simulink subsystem "active_infeed"  (R2023b)
settings: Solver=VariableStepAuto  StartTime=0.0  StopTime=10.0  RelTol=1e-3
model mask{P=0, Ts=0}
values from neighbouring files (symbols this model uses):
  Ts = ts(k)    [example_MW.m]
libraries: ee_lib x11, nesl_utility x10, fl_lib x4, eeTransforms x3, eeAdaptiveController x1, slpidlib x1, eeSinusoidalMeasurement x1, eeGeneralControl x1, eePwmGeneratorTwoLevel x1
settings Model: Creator=neugebch  LastModifiedBy=neugebch

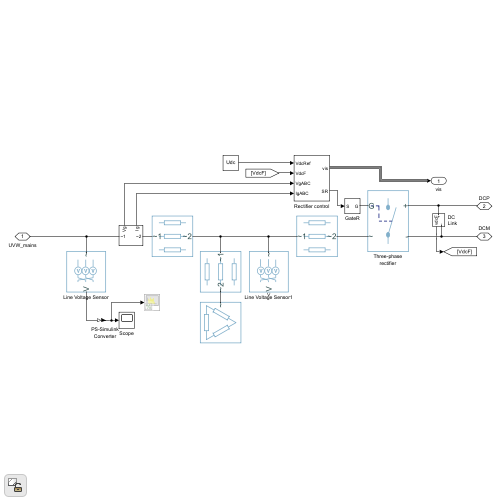
[thumbnail: Simulink's stored preview of the top-level diagram]
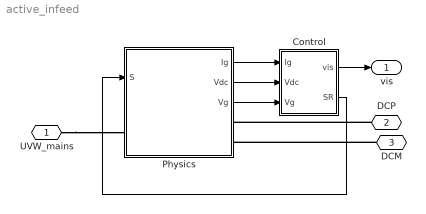
== system active_infeed ==
  Control : Subsystem
  Physics : Subsystem
  UVW_mains : PMIOPort  Side=Left
  DCP : PMIOPort  Port=2  Side=Right
  DCM : PMIOPort  Port=3  Side=Right
  vis : Outport
  wires:
  Physics/3(Vg) -> Control/3(Vg)
  Physics/2(Vdc) -> Control/2(Vdc)
  Physics/1(Ig) -> Control/1(Ig)
  Control/2(SR) -> Physics/1(S)
  Control/1(vis) -> vis/1
  connections:
  DCM/RConn1 -- Physics/RConn2
  UVW_mains/RConn1 -- Physics/LConn1
  DCP/RConn1 -- Physics/RConn1

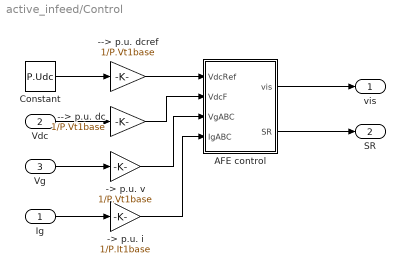
== system active_infeed/Control ==
  Ig : Inport
  Vdc : Inport  Port=2
  Vg : Inport  Port=3
  --> p.u. dc : Gain  Gain=1/P.Vt1base
  --> p.u. dcref : Gain  Gain=1/P.Vt1base
  -> p.u. i : Gain  Gain=1/P.It1base
  -> p.u. v : Gain  Gain=1/P.Vt1base
  AFE control : Subsystem
  Constant : Constant  Value=P.Udc
  vis : Outport
  SR : Outport  Port=2
  wires:
  --> p.u. dc/1 -> AFE control/2(VdcF)
  Vdc/1 -> --> p.u. dc/1
  --> p.u. dcref/1 -> AFE control/1(VdcRef)
  AFE control/2(SR) -> SR/1
  Ig/1 -> -> p.u. i/1
  AFE control/1(vis) -> vis/1
  Vg/1 -> -> p.u. v/1
  Constant/1 -> --> p.u. dcref/1
  -> p.u. v/1 -> AFE control/3(VgABC)
  -> p.u. i/1 -> AFE control/4(IgABC)

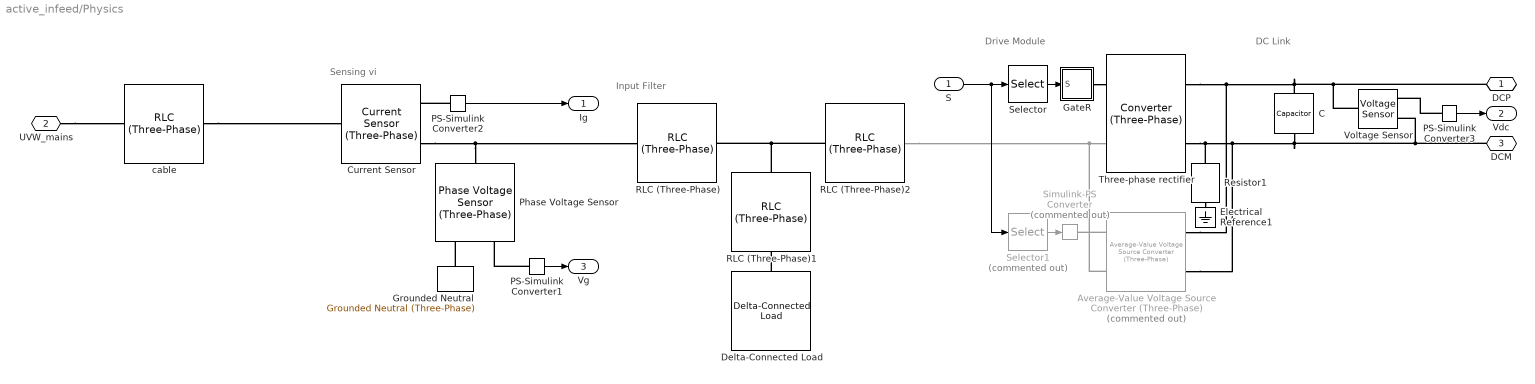
== system active_infeed/Physics ==
  note: Sensing vi
  note: Input Filter
  note: DC
      | Link
  note: Drive Module
  S : Inport
  Average-Value Voltage Source Converter (Three-Phase) : ee_lib/Semiconductors & Converters/Converters/Average-Value Voltage Source Converter (Three-Phase)  Commented=on  port_option=ee.enum.threePhasePort.composite  frequency_option=ee.enum.converters.frequency.constant  FRated=P.fn Hz  losses_parameterization=ee.enum.converters.losses.fixed  Pfixed=1 W  ks=0.01  kc1=1.7 V  kc2=0.01 Ohm  Ploss_vect=[100, 800, 1870, 3250, 4900] W  Irms_vect=[10, 100, 200, 300, 400] A  Vdc_nom=300 V  thermal_mass=30000 J/K  temperature_specify=off  temperature_priority=High  temperature=298.15 K  temperature_nominal_specify=off  temperature_nominal_unit=K  temperature_nominal_value=1
      settings: InternalSimscapePortConfiguration="{\"Bottom\":[],\"Left\":[{\"id\":\"ModWave\",\"label\":\"ModWave\",\"type\":\"input\"},{\"id\":\"N\",\"label\":\"~\",\"type\":\"foundation.electrical.three_phase\"}],\"Right\":[{\"id\":\"p\",\"label\":\"+\",\"type\":\"foundation.electrical.electrical\"},{\"id\":\"n\",\"label\":\"-\",\"type\":\"foundation.electrical.electrical\"}],\"Top\":[]}"
  C : fl_lib/Electrical/Electrical Elements/Capacitor  c=P.Cd F  r=P.Rd Ohm  g=1/P.Rd2 1/Ohm  i_specify=off  i_priority=None  i=0 A  i_nominal_specify=off  i_nominal_unit=A  i_nominal_value=1  v_specify=off  v_priority=None  v=0 V  v_nominal_specify=off  v_nominal_unit=V  v_nominal_value=1  vc_specify=on  vc_priority=None  vc=0 V  vc_nominal_specify=off  vc_nominal_unit=V  vc_nominal_value=1
  Current Sensor : ee_lib/Sensors & Transducers/Current Sensor (Three-Phase)
  Delta-Connected Load : ee_lib/Passive/RLC Assemblies/Delta-Connected Load  parameterization=ee.enum.rlc.parameterization.direct  component_structure=ee.enum.rlc.structure.C  component_structure_PQ=ee.enum.rlc.structure.SeriesRC  R=1 Ohm  L=1e-3 H  C=P.Cz F  VRated=24e3 V  FRated=60 Hz  P=1e3 W  Qpos=1e2 A*V  Qneg=-1e2 A*V  R_parasitic=0 Ohm  G_parasitic=0 1/Ohm  R_parasitic_PQ=0 Ohm  G_parasitic_PQ=0 1/Ohm  Vmag0=24e3 V  Vang0=0 deg  Freq0=60 Hz  IL_specify=off  IL_priority=High  IL=[0, 0, 0] A  IL_nominal_specify=off  IL_nominal_unit=A  IL_nominal_value=1  VC_specify=off  VC_priority=High  VC=[0, 0, 0] V  VC_nominal_specify=off  VC_nominal_unit=V  VC_nominal_value=1
      settings: InternalSimscapePortConfiguration="{\"Bottom\":[],\"Left\":[{\"id\":\"N\",\"label\":\"~\",\"type\":\"foundation.electrical.three_phase\"}],\"Right\":[],\"Top\":[]}"
  Electrical Reference1 : fl_lib/Electrical/Electrical Elements/Electrical Reference
  GateR : Subsystem
  Grounded Neutral : ee_lib/Connectors & References/Grounded Neutral (Three-Phase)
  PS-Simulink Converter1 : nesl_utility/PS-Simulink Converter  PhysicalDomain=network_engine_domain  SubClassName=ps_output  LeftPortType=input  RightPortType=output  PseudoPeriodic=off  Frequencies=[]  VectorFormat=1-D array  Unit=1  AffineConversion=off
  PS-Simulink Converter2 : nesl_utility/PS-Simulink Converter  PhysicalDomain=network_engine_domain  SubClassName=ps_output  LeftPortType=input  RightPortType=output  PseudoPeriodic=off  Frequencies=[]  VectorFormat=1-D array  Unit=1  AffineConversion=off
  PS-Simulink Converter3 : nesl_utility/PS-Simulink Converter  PhysicalDomain=network_engine_domain  SubClassName=ps_output  LeftPortType=input  RightPortType=output  PseudoPeriodic=off  Frequencies=[]  VectorFormat=1-D array  Unit=1  AffineConversion=off
  Phase Voltage Sensor : ee_lib/Sensors & Transducers/Phase Voltage Sensor (Three-Phase)
  RLC (Three-Phase) : ee_lib/Passive/RLC Assemblies/RLC (Three-Phase)  component_structure=ee.enum.rlc.structure.SeriesRL  R=P.Le*P.om/P.X_R_Le Ohm  L=P.Le H  C=1e-6 F  R_parasitic=0 Ohm  G_parasitic=0 1/Ohm  IL_specify=off  IL_priority=High  IL=[0, 0, 0] A  IL_nominal_specify=off  IL_nominal_unit=A  IL_nominal_value=1  VC_specify=off  VC_priority=High  VC=[0, 0, 0] V  VC_nominal_specify=off  VC_nominal_unit=V  VC_nominal_value=1
      settings: InternalSimscapePortConfiguration="{\"Bottom\":[],\"Left\":[{\"id\":\"N1\",\"label\":\"~1\",\"type\":\"foundation.electrical.three_phase\"}],\"Right\":[{\"id\":\"N2\",\"label\":\"~2\",\"type\":\"foundation.electrical.three_phase\"}],\"Top\":[]}"
  RLC (Three-Phase)1 : ee_lib/Passive/RLC Assemblies/RLC (Three-Phase)  component_structure=ee.enum.rlc.structure.R  R=P.Rz Ohm  L=1e-3 H  C=1e-6 F  R_parasitic=0 Ohm  G_parasitic=0 1/Ohm  IL_specify=off  IL_priority=High  IL=[0, 0, 0] A  IL_nominal_specify=off  IL_nominal_unit=A  IL_nominal_value=1  VC_specify=off  VC_priority=High  VC=[0, 0, 0] V  VC_nominal_specify=off  VC_nominal_unit=V  VC_nominal_value=1
      settings: InternalSimscapePortConfiguration="{\"Bottom\":[],\"Left\":[{\"id\":\"N1\",\"label\":\"~1\",\"type\":\"foundation.electrical.three_phase\"}],\"Right\":[{\"id\":\"N2\",\"label\":\"~2\",\"type\":\"foundation.electrical.three_phase\"}],\"Top\":[]}"
  RLC (Three-Phase)2 : ee_lib/Passive/RLC Assemblies/RLC (Three-Phase)  component_structure=ee.enum.rlc.structure.SeriesRL  R=P.Lk*P.om/P.X_R_Lk Ohm  L=P.Lk H  C=1e-6 F  R_parasitic=0 Ohm  G_parasitic=0 1/Ohm  IL_specify=off  IL_priority=High  IL=[0, 0, 0] A  IL_nominal_specify=off  IL_nominal_unit=A  IL_nominal_value=1  VC_specify=off  VC_priority=High  VC=[0, 0, 0] V  VC_nominal_specify=off  VC_nominal_unit=V  VC_nominal_value=1
      settings: InternalSimscapePortConfiguration="{\"Bottom\":[],\"Left\":[{\"id\":\"N1\",\"label\":\"~1\",\"type\":\"foundation.electrical.three_phase\"}],\"Right\":[{\"id\":\"N2\",\"label\":\"~2\",\"type\":\"foundation.electrical.three_phase\"}],\"Top\":[]}"
  Resistor1 : fl_lib/Electrical/Electrical Elements/Resistor  R=1e5 Ohm  i_specify=off  i_priority=None  i=0 A  i_nominal_specify=off  i_nominal_unit=A  i_nominal_value=1  v_specify=off  v_priority=None  v=0 V  v_nominal_specify=off  v_nominal_unit=V  v_nominal_value=1
  Selector : Selector  InputPortWidth=9  IndexOptions=Index vector (dialog)  Indices=1:6  OutputSizes=1
  Selector1 : Selector  Commented=on  InputPortWidth=9  IndexOptions=Index vector (dialog)  Indices=7:9  OutputSizes=1
  Simulink-PS Converter : nesl_utility/Simulink-PS Converter  Commented=on  PhysicalDomain=network_engine_domain  SubClassName=ps_input  LeftPortType=input  RightPortType=output  PseudoPeriodic=off  Frequencies=[]  NoiseDistribution=none  NoiseParameters=[]  Unit=1  AffineConversion=off  FilteringAndDerivatives=provide  SimscapeFilterOrder=1  InputFilterTimeConstant=0.001  UdotUserProvided=0
  Three-phase rectifier : ee_lib/Semiconductors & Converters/Converters/Converter (Three-Phase)  port_option=ee.enum.threePhasePort.composite  device_type=ee.enum.converters.switchingdevice.ideal  K=0  Vf=0.8 V  Ron=0.001 Ohm  Rds=0.001 Ohm  Goff=1e-5 1/Ohm  Vgt=1 V  Vgt_off=-1 V  Ih=1 A  Vth=0.5 V  diode_param=ee.enum.converters.protectiondiode.nodynamics  diode_Vf=0.8 V  diode_Ron=0.001 Ohm  diode_Goff=1e-5 1/Ohm  diode_C=50 nF  diode_iRM=-235 A  diode_iF=300 A  diode_idot=-50 A/us  diode_trr_param=ee.enum.converters.diodetrr.trr_factor  diode_trr_factor=3  diode_trr=15 us  diode_Qrr=1.5e+3 s*uA  snubber_type=ee.enum.converters.snubber.exclude  Cs=1e-5 F  Rs=1e-3 Ohm
  Voltage Sensor : fl_lib/Electrical/Electrical Sensors/Voltage Sensor
  cable : ee_lib/Passive/RLC Assemblies/RLC (Three-Phase)  component_structure=ee.enum.rlc.structure.SeriesRL  R=P.cab.l*P.cab.rl Ohm  L=P.cab.l*P.cab.ll H  C=1e-6 F  R_parasitic=0 Ohm  G_parasitic=0 1/Ohm  IL_specify=off  IL_priority=High  IL=[0, 0, 0] A  IL_nominal_specify=off  IL_nominal_unit=A  IL_nominal_value=1  VC_specify=off  VC_priority=High  VC=[0, 0, 0] V  VC_nominal_specify=off  VC_nominal_unit=V  VC_nominal_value=1
      settings: InternalSimscapePortConfiguration="{\"Bottom\":[],\"Left\":[{\"id\":\"N1\",\"label\":\"~1\",\"type\":\"foundation.electrical.three_phase\"}],\"Right\":[{\"id\":\"N2\",\"label\":\"~2\",\"type\":\"foundation.electrical.three_phase\"}],\"Top\":[]}"
  DCP : PMIOPort  Side=Right
  UVW_mains : PMIOPort  Port=2  Side=Left
  DCM : PMIOPort  Port=3  Side=Right
  Ig : Outport
  Vdc : Outport  Port=2
  Vg : Outport  Port=3
  wires:
  Selector1/1 -> Simulink-PS Converter/1
  Selector/1 -> GateR/1(S)
  PS-Simulink Converter3/1 -> Vdc/1
  PS-Simulink Converter2/1 -> Ig/1
  PS-Simulink Converter1/1 -> Vg/1
  S/1 -> Selector/1, Selector1/1
  connections:
  cable/RConn1 -- Current Sensor/LConn1
  Average-Value Voltage Source Converter (Three-Phase)/LConn1 -- Simulink-PS Converter/RConn1
  Resistor1/RConn1 -- Electrical Reference1/LConn1
  UVW_mains/RConn1 -- cable/LConn1
  PS-Simulink Converter3/LConn1 -- Voltage Sensor/RConn1
  Average-Value Voltage Source Converter (Three-Phase)/LConn2 -- Three-phase rectifier/LConn2 -- RLC (Three-Phase)2/RConn1
  GateR/RConn1 -- Three-phase rectifier/LConn1
  DCP/RConn1 -- Voltage Sensor/LConn1 -- C/LConn1 -- Average-Value Voltage Source Converter (Three-Phase)/RConn1 -- Three-phase rectifier/RConn1
  RLC (Three-Phase)/RConn1 -- RLC (Three-Phase)1/LConn1 -- RLC (Three-Phase)2/LConn1
  Phase Voltage Sensor/LConn1 -- RLC (Three-Phase)/LConn1 -- Current Sensor/RConn2
  PS-Simulink Converter2/LConn1 -- Current Sensor/RConn1
  Voltage Sensor/RConn2 -- DCM/RConn1 -- C/RConn1 -- Average-Value Voltage Source Converter (Three-Phase)/RConn2 -- Resistor1/LConn1 -- Three-phase rectifier/RConn2
  Grounded Neutral/LConn1 -- Phase Voltage Sensor/RConn2
  PS-Simulink Converter1/LConn1 -- Phase Voltage Sensor/RConn1
  Delta-Connected Load/LConn1 -- RLC (Three-Phase)1/RConn1

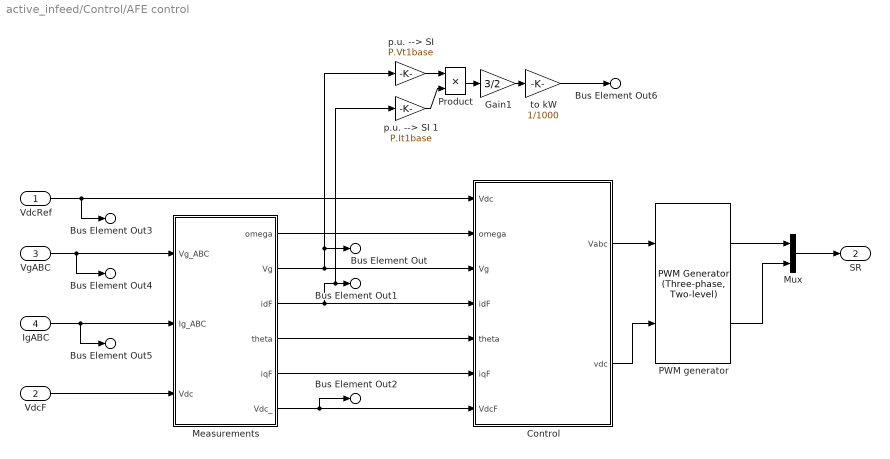
== system active_infeed/Control/AFE control ==
  VdcRef : Inport
  VdcF : Inport  Port=2
  VgABC : Inport  Port=3
  IgABC : Inport  Port=4
  Control : Subsystem
  Gain1 : Gain  Gain=3/2
  Measurements : Subsystem
  Mux : Mux  Inputs=2
  PWM generator : eePwmGeneratorTwoLevel/PWM Generator (Three-phase, Two-level)  PWMMode=Continuous PWM (CPWM)  CPWMMode=SVM: space vector modulation  DPWMMode=60 DPWM: 60 degree discontinuous PWM  fsw=P.fsw  Ts=Ts
  Product : Product
  p.u. --> SI : Gain  Gain=P.Vt1base
  p.u. --> SI 1 : Gain  Gain=P.It1base
  to kW : Gain  Gain=1/1000
  Bus Element Out : Outport  PortName=vis  Element=Vg
  Bus Element Out1 : Outport  PortName=vis  Element=idF
  Bus Element Out2 : Outport  PortName=vis  Element=VdcF
  Bus Element Out3 : Outport  PortName=vis  Element=VdcRef
  Bus Element Out4 : Outport  PortName=vis  Element=VgABC
  Bus Element Out5 : Outport  PortName=vis  Element=IgABC
  Bus Element Out6 : Outport  PortName=vis  Element=Pt
  SR : Outport  Port=2  VectorParamsAs1DForOutWhenUnconnected=off
  wires:
  Mux/1 -> SR/1
  PWM generator/1 -> Mux/1
  Control/2(vdc) -> PWM generator/2
  Control/1(Vabc) -> PWM generator/1
  PWM generator/2 -> Mux/2
  Measurements/6(Vdc_) -> Control/7(VdcF), Bus Element Out2/1
  VdcF/1 -> Measurements/3(Vdc)
  to kW/1 -> Bus Element Out6/1
  Measurements/3(idF) -> Control/4(idF), Bus Element Out1/1, p.u. --> SI 1/1
  Gain1/1 -> to kW/1
  p.u. --> SI/1 -> Product/1
  p.u. --> SI 1/1 -> Product/2
  Product/1 -> Gain1/1
  Measurements/2(Vg) -> Control/3(Vg), p.u. --> SI/1, Bus Element Out/1
  VdcRef/1 -> Bus Element Out3/1, Control/1(Vdc)
  Measurements/5(iqF) -> Control/6(iqF)
  Measurements/4(theta) -> Control/5(theta)
  Measurements/1(omega) -> Control/2(omega)
  IgABC/1 -> Measurements/2(Ig_ABC), Bus Element Out5/1
  VgABC/1 -> Measurements/1(Vg_ABC), Bus Element Out4/1

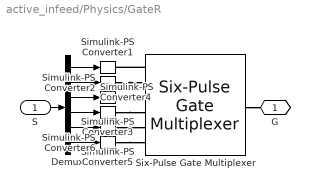
== system active_infeed/Physics/GateR ==
  S : Inport
  Demux : Demux  Outputs=6
  Simulink-PS Converter{1..6} (6 alike) : nesl_utility/Simulink-PS Converter  PhysicalDomain=network_engine_domain  SubClassName=ps_input  LeftPortType=input  RightPortType=output  PseudoPeriodic=off  Frequencies=[]  NoiseDistribution=none  NoiseParameters=[]  Unit=1  AffineConversion=off  FilteringAndDerivatives=zero  SimscapeFilterOrder=1  InputFilterTimeConstant=0.001  UdotUserProvided=1
  Six-Pulse Gate Multiplexer : ee_lib/Semiconductors & Converters/Converters/Six-Pulse Gate Multiplexer  port_option=ee.enum.controlport.ps
  G : PMIOPort  Side=Right
  wires:
  Demux/3 -> Simulink-PS Converter3/1
  Demux/6 -> Simulink-PS Converter6/1
  Demux/5 -> Simulink-PS Converter5/1
  S/1 -> Demux/1
  Demux/2 -> Simulink-PS Converter2/1
  Demux/1 -> Simulink-PS Converter1/1
  Demux/4 -> Simulink-PS Converter4/1
  connections:
  Six-Pulse Gate Multiplexer/RConn1 -- G/RConn1
  Six-Pulse Gate Multiplexer/LConn1 -- Simulink-PS Converter1/RConn1
  Simulink-PS Converter5/RConn1 -- Six-Pulse Gate Multiplexer/LConn5
  Simulink-PS Converter6/RConn1 -- Six-Pulse Gate Multiplexer/LConn6
  Simulink-PS Converter3/RConn1 -- Six-Pulse Gate Multiplexer/LConn3
  Simulink-PS Converter2/RConn1 -- Six-Pulse Gate Multiplexer/LConn2
  Simulink-PS Converter4/RConn1 -- Six-Pulse Gate Multiplexer/LConn4

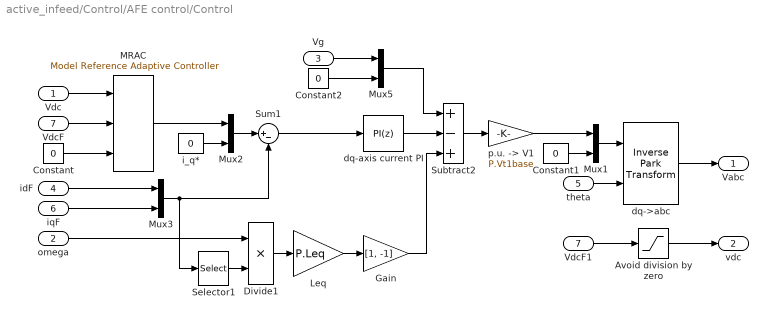
== system active_infeed/Control/AFE control/Control ==
  Vdc : Inport
  omega : Inport  Port=2
  Vg : Inport  Port=3
  idF : Inport  Port=4
  theta : Inport  Port=5
  iqF : Inport  Port=6
  VdcF : Inport  Port=7
  Avoid division by zero : Saturate  UpperLimit=1e6  LowerLimit=10
  Constant : Constant  Value=0
  Constant1 : Constant  Value=0  SampleTime=P.Tsc
  Constant2 : Constant  Value=0
  Divide1 : Product  Inputs=**
  Gain : Gain  Gain=[1, -1]
  Leq : Gain  Gain=P.Leq
  MRAC : eeAdaptiveController/Model Reference Adaptive Controller  Kp=P.Kp_vdc  Ki=P.Ki_vdc  Kd=0  Kaw=1000  UseFilter=off  N=100  up=5  lo=-5  Ts=P.Tsc  TfType=Discrete-time  numd=P.numd  dend=P.dend  numc=[1 1]  denc=[1 2 1]  Tsd=0.01  gamma=0.8
  Mux{1..3,5} (4 alike) : Mux  Inputs=2
  Selector1 : Selector  InputPortWidth=2  IndexOptions=Index vector (dialog)  Indices=[2 1]  OutputSizes=1
  Subtract2 : Sum  Inputs=+-+
  Sum1 : Sum  Inputs=|+-
  VdcF1 : InportShadow  Port=7
  dq->abc : eeTransforms/Inverse Park Transform  AxisAlignment=Q-axis  PowerInvariant=off
  dq-axis current PI : slpidlib/PID Controller  Controller=PI  Form=Parallel  TimeDomain=Discrete-time  UseExternalTs=off  SampleTime=P.Tsc  IntegratorMethod=Forward Euler  FilterMethod=Forward Euler  ControllerParametersSource=internal  P=[P.Kp_id, P.Kp_iq]  I=[P.Ki_id, P.Ki_iq]  UseKiTs=off  D=0  N=100  UseFilter=on  TunerSelectOption=Transfer Function Based (PID Tuner App)  InitialConditionSource=internal  InitialConditionForIntegrator=0  InitialConditionForFilter=0  DifferentiatorICPrevScaledInput=0  ExternalReset=none  TrackingMode=off  Kt=1  LimitOutput=on  SatLimitsSource=internal  UpperSaturationLimit=P.Req*1*10  LowerSaturationLimit=-P.Req*1*10  LinearizeAsGain=on  AntiWindupMode=back-calculation  Kb=1000  LimitIntegrator=off  UpperIntegratorSaturationLimit=inf  LowerIntegratorSaturationLimit=-inf  POutMin=[]  POutMax=[]  IOutMin=[]  IOutMax=[]  DOutMin=[]  DOutMax=[]  NOutMin=[]  NOutMax=[]  SumOutMin=[]  SumOutMax=[]  SaturationOutMin=[]  SaturationOutMax=[]  PParamMin=[]  PParamMax=[]  IParamMin=[]  IParamMax=[]  DParamMin=[]  DParamMax=[]  NParamMin=[]  NParamMax=[]  KbParamMin=[]  KbParamMax=[]  KtParamMin=[]  KtParamMax=[]  KbOutMin=[]  KbOutMax=[]  KtOutMin=[]  KtOutMax=[]  IntegratorOutMin=[]  IntegratorOutMax=[]  FilterOutMin=[]  FilterOutMax=[]  SumI1OutMin=[]  SumI1OutMax=[]  SumI2OutMin=[]  SumI2OutMax=[]  SumI3OutMin=[]  SumI3OutMax=[]  SumI4OutMin=[]  SumI4OutMax=[]  SumDOutMin=[]  SumDOutMax=[]  DifferentiatorOutMin=[]  DifferentiatorOutMax=[]  FilterDiffOutCoefMin=[]  FilterDiffOutCoefMax=[]  ReciprocalOutMin=[]  ReciprocalOutMax=[]  SumDenOutMin=[]  SumDenOutMax=[]  SumNumOutMin=[]  SumNumOutMax=[]  DivideOutMin=[]  DivideOutMax=[]  UdiffTsProdOutMin=[]  UdiffTsProdOutMax=[]  NTsProdOutMin=[]  NTsProdOutMax=[]  UintegralTsProdOutMin=[]  UintegralTsProdOutMax=[]  UngainTsProdOutMin=[]  UngainTsProdOutMax=[]  ClampingZeroOutDataTypeStr=Inherit: Inherit via back propagation  ClampingZeroOutMin=[]  ClampingZeroOutMax=[]  FilterDenConstantOutDataTypeStr=Inherit: Inherit via back propagation  FilterDenConstantOutMin=[]  FilterDenConstantOutMax=[]  PCopyOutDataTypeStr=Inherit: Inherit via back propagation  PCopyOutMin=[]  PCopyOutMax=[]  NCopyOutDataTypeStr=Inherit: Inherit via back propagation  NCopyOutMin=[]  NCopyOutMax=[]  IntegratorContinuousStateAttributes=''  IntegratorStateMustResolveToSignalObject=off  IntegratorRTWStateStorageClass=Auto  FilterContinuousStateAttributes=''  FilterStateMustResolveToSignalObject=off  FilterRTWStateStorageClass=Auto  ParallelPVariant=InternalParameters  IdealPVariant=Disabled  IVariant=InternalParameters  DVariant=Disabled  IntegratorVariant=Discrete  SatVariant=Enabled  AWVariant=BackCalculation  PCopyVariant=Disabled  TRVariant=Disabled  FdbkBlocksVariant=Forward  IdealPFdbkVariant=Disabled  SatFdbkVariant=Disabled  DerivativeFilterVariant=Disabled  NVariant=Disabled  NCopyVariant=Disabled_SignalSpec  FilterICVariant=Disabled  IntegratorICVariant=InternalICs  ExternalResetVariant=Disabled  TRSumVariant=Passthrough  SumFdbkVariant=Disabled  SumVariant=Sum_PI  TsampFilterVariant=InternalTs  TsampNgainVariant=Passthrough  TsampIntegralVariant=Disabled_SignalSpec  ExternalSaturationOutDataTypeStr=Inherit: Same as second input
  i_q* : Constant  Value=0
  "p.u. -> V1" : Gain  Gain=P.Vt1base
  Vabc : Outport
  vdc : Outport  Port=2
  wires:
  "p.u. -> V1"/1 -> Mux1/1
  Selector1/1 -> Divide1/2
  Gain/1 -> Subtract2/3
  Constant2/1 -> Mux5/2
  Mux5/1 -> Subtract2/1
  Vg/1 -> Mux5/1
  dq-axis current PI/1 -> Subtract2/2
  Sum1/1 -> dq-axis current PI/1
  Mux3/1 -> Selector1/1, Sum1/2
  Mux2/1 -> Sum1/1
  Leq/1 -> Gain/1
  Divide1/1 -> Leq/1
  MRAC/1 -> Mux2/1
  Constant/1 -> MRAC/3
  VdcF/1 -> MRAC/2
  Vdc/1 -> MRAC/1
  VdcF1/1 -> Avoid division by zero/1
  iqF/1 -> Mux3/2
  dq->abc/1 -> Vabc/1
  idF/1 -> Mux3/1
  Constant1/1 -> Mux1/2
  Mux1/1 -> dq->abc/1
  Subtract2/1 -> "p.u. -> V1"/1
  omega/1 -> Divide1/1
  i_q*/1 -> Mux2/2
  Avoid division by zero/1 -> vdc/1
  theta/1 -> dq->abc/2

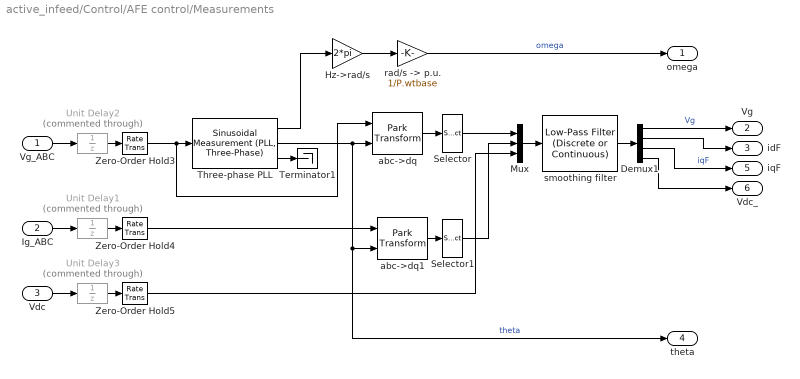
== system active_infeed/Control/AFE control/Measurements ==
  Vg_ABC : Inport
  Ig_ABC : Inport  Port=2
  Vdc : Inport  Port=3
  Demux1 : Demux
  Hz->rad/s : Gain  Gain=2*pi
  Mux : Mux  Inputs=3
  Selector : Selector  InputPortWidth=3  IndexOptions=Index vector (dialog)  Indices=[1]  OutputSizes=1
  Selector1 : Selector  InputPortWidth=3  IndexOptions=Index vector (dialog)  Indices=[1 2]  OutputSizes=1
  Terminator1 : Terminator
  Three-phase PLL : eeSinusoidalMeasurement/Sinusoidal Measurement (PLL, Three-Phase)  Kp_LF=45  Ki_LF=1250  F0=fn  Theta0=0  Ts=P.Tsc
  Unit Delay1 : UnitDelay  Commented=through  SampleTime=Ts  HasFrameUpgradeWarning=on
  Unit Delay2 : UnitDelay  Commented=through  SampleTime=Ts  HasFrameUpgradeWarning=on
  Unit Delay3 : UnitDelay  Commented=through  SampleTime=Ts  HasFrameUpgradeWarning=on
  Zero-Order Hold3 : RateTransition  OutPortSampleTime=P.Tsc
  Zero-Order Hold4 : RateTransition  OutPortSampleTime=P.Tsc
  Zero-Order Hold5 : RateTransition  OutPortSampleTime=P.Tsc
  abc->dq : eeTransforms/Park Transform  AxisAlignment=Q-axis  PowerInvariant=off
  abc->dq1 : eeTransforms/Park Transform  AxisAlignment=Q-axis  PowerInvariant=off
  "rad/s -> p.u." : Gain  Gain=1/P.wtbase
  smoothing filter : eeGeneralControl/Low-Pass Filter (Discrete or Continuous)  K=1  T=1e-3  B=inf  A=-inf  init_option=Inherited from block input  x0=0  Ts=P.Tsc
  omega : Outport  VectorParamsAs1DForOutWhenUnconnected=off
  Vg : Outport  Port=2  VectorParamsAs1DForOutWhenUnconnected=off
  idF : Outport  Port=3  VectorParamsAs1DForOutWhenUnconnected=off
  theta : Outport  Port=4  VectorParamsAs1DForOutWhenUnconnected=off
  iqF : Outport  Port=5  VectorParamsAs1DForOutWhenUnconnected=off
  Vdc_ : Outport  Port=6  VectorParamsAs1DForOutWhenUnconnected=off
  wires:
  smoothing filter/1 -> Demux1/1
  Mux/1 -> smoothing filter/1
  Demux1/4 -> Vdc_/1
  Vdc/1 -> Unit Delay3/1
  Zero-Order Hold5/1 -> Mux/3
  Unit Delay3/1 -> Zero-Order Hold5/1
  Demux1/3 -> iqF/1  "iqF"
  "rad/s -> p.u."/1 -> omega/1  "omega"
  Vg_ABC/1 -> Unit Delay2/1
  abc->dq1/1 -> Selector1/1
  Selector1/1 -> Mux/2
  Unit Delay2/1 -> Zero-Order Hold3/1
  Zero-Order Hold4/1 -> abc->dq1/1
  Demux1/1 -> Vg/1  "Vg"
  Ig_ABC/1 -> Unit Delay1/1
  Three-phase PLL/3 -> Terminator1/1
  Selector/1 -> Mux/1
  Three-phase PLL/1 -> Hz->rad/s/1
  Zero-Order Hold3/1 -> Three-phase PLL/1, abc->dq/1
  Demux1/2 -> idF/1
  Three-phase PLL/2 -> abc->dq/2, theta/1, abc->dq1/2  "theta"
  Hz->rad/s/1 -> "rad/s -> p.u."/1
  abc->dq/1 -> Selector/1
  Unit Delay1/1 -> Zero-Order Hold4/1
